simulink model "Full_model_v1"  (R2023b)
settings: Solver=VariableStepAuto  StartTime=0.0  StopTime=simu.duration  FixedStep=simu.timestep  MaxStep=0.1  MinStep=1e-16  RelTol=1e-3
undefined symbols (not defined in the file or in its folder): ptosim, Z_OPT_fixed
libraries: fl_lib x47, nesl_utility x42, ee_lib x11, simulink x1
settings Model: Creator=tedbrekken  LastModifiedBy=inyongkim
settings DebuggingCC: UnconnectedInputMsg=warning  UnconnectedOutputMsg=warning  UnconnectedLineMsg=warning
settings ModelReferenceCC: EnableRefExpFcnMdlSchedulingChecks=on
settings RTWCC: DLArmComputeVersion=19.05

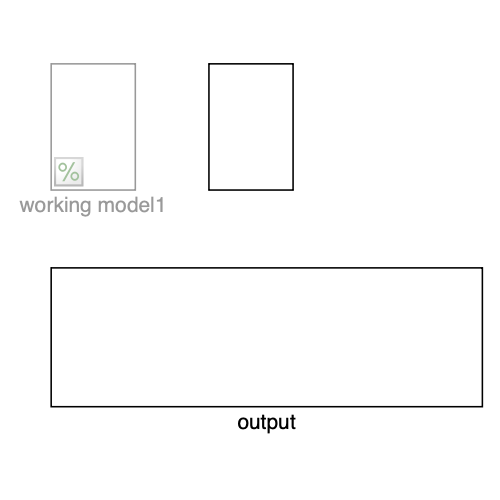
[thumbnail: Simulink's stored preview of the top-level diagram]
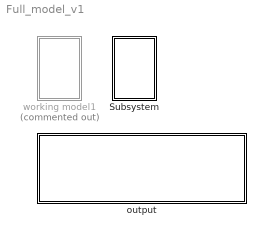
== system Full_model_v1 ==
  Subsystem : Subsystem
  output : Subsystem
  working model1 : Subsystem  Commented=on

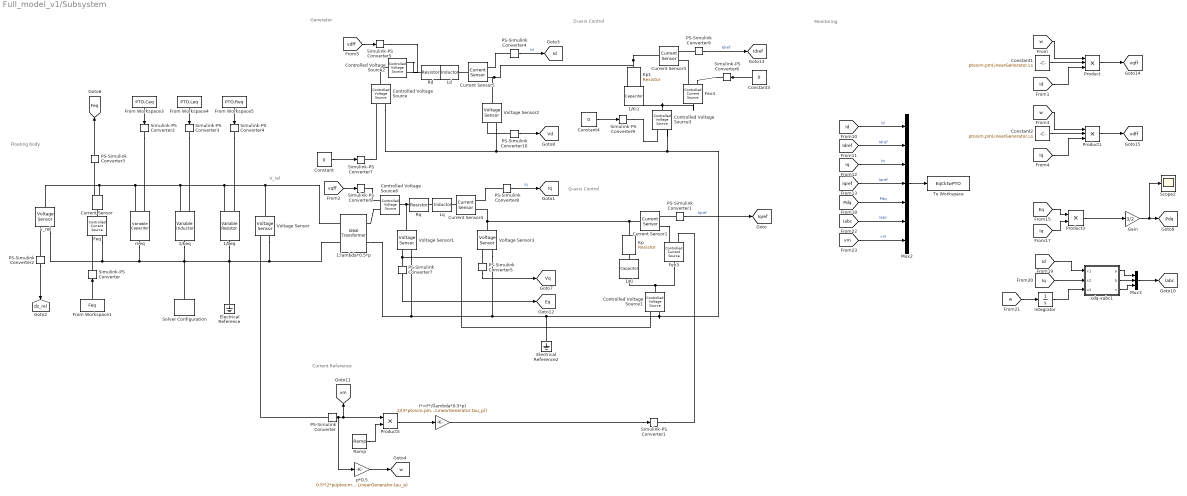
== system Full_model_v1/Subsystem ==
  note: Q-axis Control
  note: Current Reference
  note: Monitoring
  note: Generator
  note: V_rel
  note: D-axis Control
  note: Floating body
  1/Ki : fl_lib/Electrical/Electrical Elements/Capacitor  c=1/(ptosim.pmLinearGenerator.Rs*ptosim.pmLinearGenerator.BWi) F  r=1e-6 Ohm  g=0 1/Ohm  i_specify=off  i_priority=None  i=0 A  i_nominal_specify=off  i_nominal_unit=A  i_nominal_value=1  v_specify=off  v_priority=None  v=0 V  v_nominal_specify=off  v_nominal_unit=V  v_nominal_value=1  vc_specify=off  vc_priority=High  vc=0 V  vc_nominal_specify=off  vc_nominal_unit=V  vc_nominal_value=1
  1/Ki1 : fl_lib/Electrical/Electrical Elements/Capacitor  c=1/(ptosim.pmLinearGenerator.Rs*ptosim.pmLinearGenerator.BWi) F  r=1e-6 Ohm  g=0 1/Ohm  i_specify=off  i_priority=None  i=0 A  i_nominal_specify=off  i_nominal_unit=A  i_nominal_value=1  v_specify=off  v_priority=None  v=0 V  v_nominal_specify=off  v_nominal_unit=V  v_nominal_value=1  vc_specify=off  vc_priority=High  vc=0 V  vc_nominal_specify=off  vc_nominal_unit=V  vc_nominal_value=1
  1/beq : fl_lib/Electrical/Electrical Elements/Variable Resistor  Rmin=0 Ohm  thermalEnable=false  thermal_mass=1 J/K  i_specify=off  i_priority=None  i=0 A  i_nominal_specify=off  i_nominal_unit=A  i_nominal_value=1  v_specify=off  v_priority=None  v=0 V  v_nominal_specify=off  v_nominal_unit=V  v_nominal_value=1  T_specify=off  T_priority=None  T=300 K  T_nominal_specify=off  T_nominal_unit=K  T_nominal_value=1
  1/keq : ee_lib/Passive/Variable Inductor  prm=2  Lmin=1e-8 H  g=0 1/Ohm  i0=0 A  phi0=0 Wb
      settings: InternalSimscapePortConfiguration="{\"Bottom\":[],\"Left\":[{\"id\":\"L\",\"label\":\"L\",\"type\":\"input\"},{\"id\":\"p\",\"label\":\"+\",\"type\":\"foundation.electrical.electrical\"}],\"Right\":[{\"id\":\"n\",\"label\":\"-\",\"type\":\"foundation.electrical.electrical\"}],\"Top\":[]}"
  1:lambda*0.5*p : fl_lib/Electrical/Electrical Elements/Ideal Transformer  n=1/(ptosim.pmLinearGenerator.lambda_fd*0.5*(2*pi/ptosim.pmLinearGenerator.tau_p))  i1_specify=off  i1_priority=None  i1=0 A  i1_nominal_specify=off  i1_nominal_unit=A  i1_nominal_value=1  v1_specify=off  v1_priority=None  v1=0 V  v1_nominal_specify=off  v1_nominal_unit=V  v1_nominal_value=1  i2_specify=off  i2_priority=None  i2=0 A  i2_nominal_specify=off  i2_nominal_unit=A  i2_nominal_value=1  v2_specify=off  v2_priority=None  v2=0 V  v2_nominal_specify=off  v2_nominal_unit=V  v2_nominal_value=1
  Constant : Constant  Value=0
  Constant1 : Constant  Value=ptosim.pmLinearGenerator.Ls
  Constant2 : Constant  Value=ptosim.pmLinearGenerator.Ls
  Constant3 : Constant  Value=0
  Constant4 : Constant  Value=0
  Controlled Voltage Source{,1..3,6} (5 alike) : fl_lib/Electrical/Electrical Sources/Controlled Voltage Source
  Current Sensor{,1,3..5} (5 alike) : fl_lib/Electrical/Electrical Sensors/Current Sensor
  Electrical Reference : fl_lib/Electrical/Electrical Elements/Electrical Reference
  Electrical Reference2 : fl_lib/Electrical/Electrical Elements/Electrical Reference
  Feq : fl_lib/Electrical/Electrical Sources/Controlled Current Source
  Fex3 : fl_lib/Electrical/Electrical Sources/Controlled Current Source
  Fex4 : fl_lib/Electrical/Electrical Sources/Controlled Current Source
  From Workspace1 : FromWorkspace  VariableName=Feq
  From Workspace3 : FromWorkspace  VariableName=PTO.Ceq
  From Workspace4 : FromWorkspace  VariableName=PTO.Leq
  From Workspace5 : FromWorkspace  VariableName=PTO.Req
  Gain : Gain  Gain=3/2
  I*=F*/(lambda*0.5*p) : Gain  Gain=2/(3*ptosim.pmLinearGenerator.lambda_fd*0.5*(2*pi/ptosim.pmLinearGenerator.tau_p))
  Integrator : Integrator
  Kp : fl_lib/Electrical/Electrical Elements/Resistor  R=ptosim.pmLinearGenerator.Ls*ptosim.pmLinearGenerator.BWi Ohm  i_specify=off  i_priority=None  i=0 A  i_nominal_specify=off  i_nominal_unit=A  i_nominal_value=1  v_specify=off  v_priority=None  v=0 V  v_nominal_specify=off  v_nominal_unit=V  v_nominal_value=1
  Kp1 : fl_lib/Electrical/Electrical Elements/Resistor  R=ptosim.pmLinearGenerator.Ls*ptosim.pmLinearGenerator.BWi Ohm  i_specify=off  i_priority=None  i=0 A  i_nominal_specify=off  i_nominal_unit=A  i_nominal_value=1  v_specify=off  v_priority=None  v=0 V  v_nominal_specify=off  v_nominal_unit=V  v_nominal_value=1
  Ld : ee_lib/Passive/Inductor  l=ptosim.pmLinearGenerator.Ls H  enable_L_tol=ee.enum.toleranceApplication.none  L_tol=20  tol_distribution=ee.enum.toleranceDistribution.uniform  nSigma=4  r=0 Ohm  g=1e-9 1/Ohm  enable_operating_limits=ee.enum.enable.no  operating_limit_action=ee.enum.passive.reportOpLim.warn  max_working_current=1 A  power_rating=1 W  enable_faults=ee.enum.enable.no  fault_action=simscape.enum.assert.action.none  lambdaPercent=50  k_faulted=0.9999  turnsShort=ee.enum.passive.inductor.turnsShortOption.no  openCct=ee.enum.enable.no  groundShort=ee.enum.passive.inductor.groundShortOption.no  groundShortG=0 1/Ohm  tau_fault=1e-3 s  fault_trigger=ee.enum.faults.faultTrigger.temporal  t_fault=1 s  max_permissible_voltage=100 V  n_fail_on_voltage=1  max_permissible_current=1 A  t_fail_on_current=1 s  i_L_specify=off  i_L_priority=High  i_L=0 A  i_L_nominal_specify=off  i_L_nominal_unit=A  i_L_nominal_value=1
  Lq : ee_lib/Passive/Inductor  l=ptosim.pmLinearGenerator.Ls H  enable_L_tol=ee.enum.toleranceApplication.none  L_tol=20  tol_distribution=ee.enum.toleranceDistribution.uniform  nSigma=4  r=0 Ohm  g=1e-9 1/Ohm  enable_operating_limits=ee.enum.enable.no  operating_limit_action=ee.enum.passive.reportOpLim.warn  max_working_current=1 A  power_rating=1 W  enable_faults=ee.enum.enable.no  fault_action=simscape.enum.assert.action.none  lambdaPercent=50  k_faulted=0.9999  turnsShort=ee.enum.passive.inductor.turnsShortOption.no  openCct=ee.enum.enable.no  groundShort=ee.enum.passive.inductor.groundShortOption.no  groundShortG=0 1/Ohm  tau_fault=1e-3 s  fault_trigger=ee.enum.faults.faultTrigger.temporal  t_fault=1 s  max_permissible_voltage=100 V  n_fail_on_voltage=1  max_permissible_current=1 A  t_fail_on_current=1 s  i_L_specify=off  i_L_priority=High  i_L=0 A  i_L_nominal_specify=off  i_L_nominal_unit=A  i_L_nominal_value=1
  Mux2 : Mux  Inputs=7
  Mux3 : Mux  Inputs=3
  PS-Simulink Converter{,1,4..5,7..10} (8 alike) : nesl_utility/PS-Simulink Converter  PhysicalDomain=network_engine_domain  SubClassName=ps_output  LeftPortType=input  RightPortType=output  PseudoPeriodic=off  Frequencies=[]  VectorFormat=inherit  Unit=inherit  AffineConversion=off
  PS-Simulink Converter2 : nesl_utility/PS-Simulink Converter  PhysicalDomain=network_engine_domain  SubClassName=ps_output  LeftPortType=input  RightPortType=output  PseudoPeriodic=off  Frequencies=[]  VectorFormat=1-D array  Unit=inherit  AffineConversion=off
  PS-Simulink Converter3 : nesl_utility/PS-Simulink Converter  PhysicalDomain=network_engine_domain  SubClassName=ps_output  LeftPortType=input  RightPortType=output  PseudoPeriodic=off  Frequencies=[]  VectorFormat=1-D array  Unit=inherit  AffineConversion=off
  Product : Product  Inputs=3
  Product1 : Product  Inputs=3
  Product3 : Product
  Product5 : Product
  Ramp : simulink/Sources/Ramp  slope=0.1/(ptosim.pmLinearGenerator.R1+ptosim.pmLinearGenerator.R2)  start=35  InitialOutput=0.1/(ptosim.pmLinearGenerator.R1+ptosim.pmLinearGenerator.R2)
  Rd : fl_lib/Electrical/Electrical Elements/Resistor  R=ptosim.pmLinearGenerator.Rs Ohm  i_specify=off  i_priority=None  i=0 A  i_nominal_specify=off  i_nominal_unit=A  i_nominal_value=1  v_specify=off  v_priority=None  v=0 V  v_nominal_specify=off  v_nominal_unit=V  v_nominal_value=1
  Rq : fl_lib/Electrical/Electrical Elements/Resistor  R=ptosim.pmLinearGenerator.Rs Ohm  i_specify=off  i_priority=None  i=0 A  i_nominal_specify=off  i_nominal_unit=A  i_nominal_value=1  v_specify=off  v_priority=None  v=0 V  v_nominal_specify=off  v_nominal_unit=V  v_nominal_value=1
  Scope2 : Scope
  Simulink-PS Converter{,1..9} (10 alike) : nesl_utility/Simulink-PS Converter  PhysicalDomain=network_engine_domain  SubClassName=ps_input  LeftPortType=input  RightPortType=output  PseudoPeriodic=off  Frequencies=[]  NoiseDistribution=none  NoiseParameters=[]  Unit=1  AffineConversion=off  FilteringAndDerivatives=provide  SimscapeFilterOrder=1  InputFilterTimeConstant=0.001  UdotUserProvided=0
  Solver Configuration : nesl_utility/Solver Configuration  PhysicalDomain=network_engine_domain  SubClassName=solver  LeftPortType=input  RightPortType=generic  Tones=[]  Harmonics=[]  SimulateNoise=off  Profile=off  UseLocalSampling=off  EnableSwitchedLinearOptims=on  FrequencyDomain=off  UseCCode=off  RelTol=0.001  AbsTol=1e-06  MinStep=1e-09  ToWorkspace=off  RevertToSquareIcSolve=off  NumHomotopyIterations=100  PhasorMode=off  PhasorModeNumHarmonics=1  ConsistencySolver=NEWTON_FTOL  IndexReductionMethod=DerivativeReplacement  DoDC=off  ResidualTolerance=1e-09  ConsistencyTolSource=GLOBAL  ConsistencyAbsTol=0.001  ConsistencyRelTol=0.001  ConsistencyTolFactor=0.001  UseLocalSolver=off  LocalSolverChoice=NE_TRAPEZOIDAL_ADVANCER  ResolveIndetEquations=on  FunctionEvalNumThread=1  LocalSolverSampleTime=0.1  DoFixedCost=off  MaxNonlinIter=3  MaxModeIter=2  ComputeImpulses=off  ImpulseIterations=2  LinearAlgebra=auto  LinearAlgebraNumThread=0  EquationFormulation=NE_TIME_EF  DelaysMemoryBudget=1024  AutomaticFiltering=off  FilteringTimeConstant=0.001  PartitionStorageMethod=AS_NEEDED  PartitionMemoryBudget=1024  PartitionMethod=ROBUST  MultibodyUseLocalSolver=off  MultibodyLocalSolverChoice=ODE1  MultibodyLocalSolverSampleTime=0.001
  To Workspace : ToWorkspace  VariableName=EqCktwPTO  SaveFormat=Timeseries  SampleTime=-1
  Voltage Sensor{,1..3} (4 alike) : fl_lib/Electrical/Electrical Sensors/Voltage Sensor
  meq : ee_lib/Passive/Variable Capacitor  prm=2  Cmin=1e-9 F  r=0 Ohm  v0=0 V  q0=0 C
      settings: InternalSimscapePortConfiguration="{\"Bottom\":[],\"Left\":[{\"id\":\"C\",\"label\":\"C\",\"type\":\"input\"},{\"id\":\"p\",\"label\":\"+\",\"type\":\"foundation.electrical.electrical\"}],\"Right\":[{\"id\":\"n\",\"label\":\"-\",\"type\":\"foundation.electrical.electrical\"}],\"Top\":[]}"
  p*0.5 : Gain  Gain=0.5*(2*pi/ptosim.pmLinearGenerator.tau_p)
  v_rel : fl_lib/Electrical/Electrical Sensors/Voltage Sensor
  xdq-xabc1 : MATLAB Function  TreatAsAtomicUnit=on
  tag scope: Eq=global, Feq=global, Iabc=global, Id=global, Idref=global, Iq=global, Iqref=global, Pdq=global, Vd=global, Vq=global, dz_rel=global, vdff=global, vm=global, vqff=global, w=global
  wires:
  From Workspace3/1 -> Simulink-PS Converter2/1
  From Workspace1/1 -> Simulink-PS Converter/1
  PS-Simulink Converter2/1 -> [dz_rel]
  PS-Simulink Converter3/1 -> [Feq]
  From Workspace4/1 -> Simulink-PS Converter3/1
  From Workspace5/1 -> Simulink-PS Converter4/1
  PS-Simulink Converter/1 -> [vm], Product5/1, p*0.5/1
  [vqff] -> Simulink-PS Converter8/1
  [vdff] -> Simulink-PS Converter5/1
  PS-Simulink Converter7/1 -> [Eq]
  Ramp/1 -> Product5/2
  PS-Simulink Converter9/1 -> [Idref]  "Idref"
  Constant3/1 -> Simulink-PS Converter6/1
  PS-Simulink Converter1/1 -> [Iqref]  "Iqref"
  PS-Simulink Converter4/1 -> [Id]  "Id"
  Product5/1 -> I*=F*/(lambda*0.5*p)/1
  Constant/1 -> Simulink-PS Converter7/1
  PS-Simulink Converter10/1 -> [Vd]
  PS-Simulink Converter8/1 -> [Iq]  "Iq"
  I*=F*/(lambda*0.5*p)/1 -> Simulink-PS Converter1/1
  p*0.5/1 -> [w]
  PS-Simulink Converter5/1 -> [Vq]
  [Idref] -> Mux2/2  "Idref"
  [Iabc] -> Mux2/6  "Iabc"
  [Eq] -> Product3/1
  xdq-xabc1/3(c) -> Mux3/3
  Gain/1 -> Scope2/1, [Pdq]
  [Iqref] -> Mux2/4  "Iqref"
  Product3/1 -> Gain/1
  [w] -> Product1/1
  [Iq] -> Mux2/3  "Iq"
  [Iq] -> Product1/3
  Product/1 -> [vqff]
  xdq-xabc1/1(a) -> Mux3/1
  [Id] -> Product/3
  [Pdq] -> Mux2/5  "Pdq"
  xdq-xabc1/2(b) -> Mux3/2
  Mux3/1 -> [Iabc]
  [Id] -> xdq-xabc1/1(x1)
  [w] -> Product/1
  [Id] -> Mux2/1  "Id"
  Mux2/1 -> To Workspace/1
  Product1/1 -> [vdff]
  [Iq] -> Product3/2
  Integrator/1 -> xdq-xabc1/3(u1)
  [vm] -> Mux2/7  "vm"
  [Iq] -> xdq-xabc1/2(x2)
  Constant1/1 -> Product/2
  Constant2/1 -> Product1/2
  [w] -> Integrator/1
  Constant4/1 -> Simulink-PS Converter9/1
  connections:
  Current Sensor/RConn1 -- PS-Simulink Converter3/LConn1
  PS-Simulink Converter2/LConn1 -- v_rel/RConn1
  Simulink-PS Converter4/RConn1 -- 1/beq/LConn1
  Simulink-PS Converter/RConn1 -- Feq/RConn1
  Simulink-PS Converter3/RConn1 -- 1/keq/LConn1
  Voltage Sensor/LConn1 -- 1:lambda*0.5*p/LConn1 -- 1/beq/LConn2 -- Current Sensor/RConn2 -- v_rel/LConn1 -- meq/LConn2 -- 1/keq/LConn2
  Simulink-PS Converter2/RConn1 -- meq/LConn1
  Electrical Reference/LConn1 -- Solver Configuration/RConn1 -- v_rel/RConn2 -- Feq/RConn2 -- meq/RConn1 -- 1/keq/RConn1 -- 1:lambda*0.5*p/LConn2 -- Voltage Sensor/RConn2 -- 1/beq/RConn1
  Feq/LConn1 -- Current Sensor/LConn1
  PS-Simulink Converter7/LConn1 -- Controlled Voltage Source1/RConn1 -- Voltage Sensor1/RConn1
  PS-Simulink Converter9/LConn1 -- Current Sensor3/RConn1
  Voltage Sensor2/RConn2 -- Electrical Reference2/LConn1 -- Voltage Sensor3/RConn2 -- Voltage Sensor1/RConn2 -- 1:lambda*0.5*p/RConn2 -- Controlled Voltage Source1/RConn2 -- Controlled Voltage Source3/RConn2 -- Controlled Voltage Source/RConn2
  PS-Simulink Converter/LConn1 -- Voltage Sensor/RConn1
  Controlled Voltage Source6/LConn1 -- Voltage Sensor1/LConn1 -- Rq/LConn1
  Controlled Voltage Source2/LConn1 -- Controlled Voltage Source/LConn1
  Kp/LConn1 -- Current Sensor4/RConn2 -- Voltage Sensor3/LConn1 -- Current Sensor1/LConn1
  Kp1/LConn1 -- Voltage Sensor2/LConn1 -- Current Sensor5/RConn2 -- Current Sensor3/LConn1
  Rq/RConn1 -- Lq/LConn1
  Controlled Voltage Source3/LConn1 -- 1/Ki1/RConn1 -- Fex4/LConn1
  PS-Simulink Converter4/LConn1 -- Current Sensor5/RConn1
  PS-Simulink Converter1/LConn1 -- Current Sensor1/RConn1
  Simulink-PS Converter1/RConn1 -- Fex3/RConn1
  Simulink-PS Converter7/RConn1 -- Controlled Voltage Source/RConn1
  Simulink-PS Converter8/RConn1 -- Controlled Voltage Source6/RConn1
  Rd/RConn1 -- Ld/LConn1
  1/Ki/LConn1 -- Kp/RConn1
  PS-Simulink Converter8/LConn1 -- Current Sensor4/RConn1
  Current Sensor1/RConn2 -- Fex3/RConn2
  Controlled Voltage Source1/LConn1 -- 1/Ki/RConn1 -- Fex3/LConn1
  Current Sensor5/LConn1 -- Ld/RConn1
  PS-Simulink Converter5/LConn1 -- Voltage Sensor3/RConn1
  Current Sensor4/LConn1 -- Lq/RConn1
  Fex4/RConn2 -- Current Sensor3/RConn2
  1/Ki1/LConn1 -- Kp1/RConn1
  Simulink-PS Converter5/RConn1 -- Controlled Voltage Source2/RConn1
  Controlled Voltage Source2/RConn2 -- Rd/LConn1
  Simulink-PS Converter6/RConn1 -- Fex4/RConn1
  Controlled Voltage Source6/RConn2 -- 1:lambda*0.5*p/RConn1
  PS-Simulink Converter10/LConn1 -- Voltage Sensor2/RConn1
  Simulink-PS Converter9/RConn1 -- Controlled Voltage Source3/RConn1

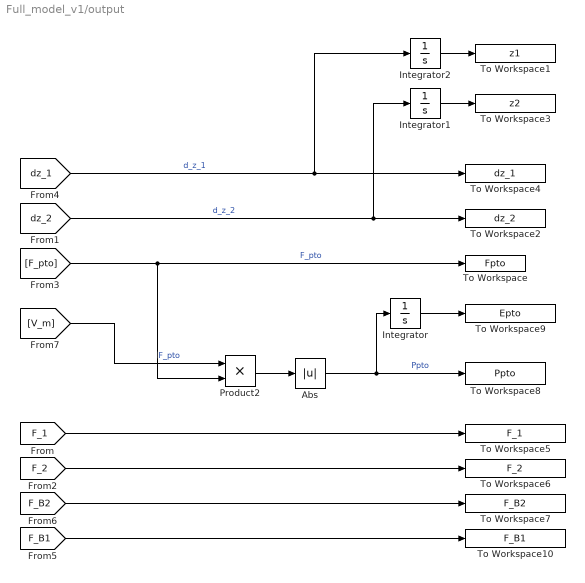
== system Full_model_v1/output ==
  Abs : Abs  SaturateOnIntegerOverflow=off
  Integrator : Integrator
  Integrator1 : Integrator
  Integrator2 : Integrator
  Product2 : Product
  To Workspace : ToWorkspace  VariableName=Fpto  SaveFormat=Timeseries  SampleTime=-1
  To Workspace1 : ToWorkspace  VariableName=z1  SaveFormat=Timeseries  SampleTime=-1
  To Workspace10 : ToWorkspace  VariableName=F_B1  SaveFormat=Timeseries  SampleTime=-1
  To Workspace2 : ToWorkspace  VariableName=dz_2  SaveFormat=Timeseries  SampleTime=-1
  To Workspace3 : ToWorkspace  VariableName=z2  SaveFormat=Timeseries  SampleTime=-1
  To Workspace4 : ToWorkspace  VariableName=dz_1  SaveFormat=Timeseries  SampleTime=-1
  To Workspace5 : ToWorkspace  VariableName=F_1  SaveFormat=Timeseries  SampleTime=-1
  To Workspace6 : ToWorkspace  VariableName=F_2  SaveFormat=Timeseries  SampleTime=-1
  To Workspace7 : ToWorkspace  VariableName=F_B2  SaveFormat=Timeseries  SampleTime=-1
  To Workspace8 : ToWorkspace  VariableName=Ppto  SaveFormat=Timeseries  SampleTime=-1
  To Workspace9 : ToWorkspace  VariableName=Epto  SaveFormat=Timeseries  SampleTime=-1
  wires:
  Integrator/1 -> To Workspace9/1
  [dz_1] -> Integrator2/1, To Workspace4/1  "d_z_1"
  [F_pto] -> To Workspace/1, Product2/2  "F_pto"
  Abs/1 -> To Workspace8/1, Integrator/1  "Ppto"
  Product2/1 -> Abs/1
  [dz_2] -> Integrator1/1, To Workspace2/1  "d_z_2"
  [F_1] -> To Workspace5/1
  [F_2] -> To Workspace6/1
  [F_B2] -> To Workspace7/1
  [F_B1] -> To Workspace10/1
  [V_m] -> Product2/1  "F_pto"
  Integrator2/1 -> To Workspace1/1
  Integrator1/1 -> To Workspace3/1

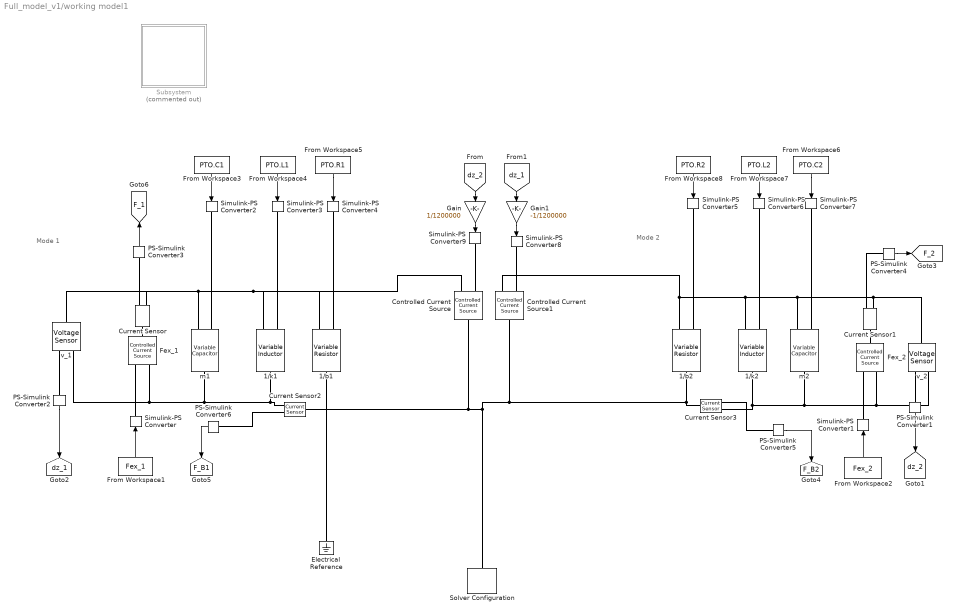
== system Full_model_v1/working model1 ==
  note: Mode 1
  note: Mode 2
  1/b1 : fl_lib/Electrical/Electrical Elements/Variable Resistor  Rmin=0 Ohm  thermalEnable=false  thermal_mass=1 J/K  i_specify=off  i_priority=None  i=0 A  i_nominal_specify=off  i_nominal_unit=A  i_nominal_value=1  v_specify=off  v_priority=None  v=0 V  v_nominal_specify=off  v_nominal_unit=V  v_nominal_value=1  T_specify=off  T_priority=None  T=300 K  T_nominal_specify=off  T_nominal_unit=K  T_nominal_value=1
  1/b2 : fl_lib/Electrical/Electrical Elements/Variable Resistor  Rmin=0 Ohm  thermalEnable=false  thermal_mass=1 J/K  i_specify=off  i_priority=None  i=0 A  i_nominal_specify=off  i_nominal_unit=A  i_nominal_value=1  v_specify=off  v_priority=None  v=0 V  v_nominal_specify=off  v_nominal_unit=V  v_nominal_value=1  T_specify=off  T_priority=None  T=300 K  T_nominal_specify=off  T_nominal_unit=K  T_nominal_value=1
  1/k1 : ee_lib/Passive/Variable Inductor  prm=2  Lmin=1e-8 H  g=0 1/Ohm  i0=0 A  phi0=0 Wb
      settings: InternalSimscapePortConfiguration="{\"Bottom\":[],\"Left\":[{\"id\":\"L\",\"label\":\"L\",\"type\":\"input\"},{\"id\":\"p\",\"label\":\"+\",\"type\":\"foundation.electrical.electrical\"}],\"Right\":[{\"id\":\"n\",\"label\":\"-\",\"type\":\"foundation.electrical.electrical\"}],\"Top\":[]}"
  1/k2 : ee_lib/Passive/Variable Inductor  prm=2  Lmin=1e-8 H  g=0 1/Ohm  i0=0 A  phi0=0 Wb
      settings: InternalSimscapePortConfiguration="{\"Bottom\":[],\"Left\":[{\"id\":\"L\",\"label\":\"L\",\"type\":\"input\"},{\"id\":\"p\",\"label\":\"+\",\"type\":\"foundation.electrical.electrical\"}],\"Right\":[{\"id\":\"n\",\"label\":\"-\",\"type\":\"foundation.electrical.electrical\"}],\"Top\":[]}"
  Controlled Current Source : fl_lib/Electrical/Electrical Sources/Controlled Current Source
  Controlled Current Source1 : fl_lib/Electrical/Electrical Sources/Controlled Current Source
  Current Sensor{,1..3} (4 alike) : fl_lib/Electrical/Electrical Sensors/Current Sensor
  Electrical Reference : fl_lib/Electrical/Electrical Elements/Electrical Reference
  Fex_1 : fl_lib/Electrical/Electrical Sources/Controlled Current Source
  Fex_2 : fl_lib/Electrical/Electrical Sources/Controlled Current Source
  From Workspace1 : FromWorkspace  VariableName=Fex_1
  From Workspace2 : FromWorkspace  VariableName=Fex_2
  From Workspace3 : FromWorkspace  VariableName=PTO.C1
  From Workspace4 : FromWorkspace  VariableName=PTO.L1
  From Workspace5 : FromWorkspace  VariableName=PTO.R1
  From Workspace6 : FromWorkspace  VariableName=PTO.C2
  From Workspace7 : FromWorkspace  VariableName=PTO.L2
  From Workspace8 : FromWorkspace  VariableName=PTO.R2
  Gain : Gain  Gain=1/1200000
  Gain1 : Gain  Gain=-1/1200000
  PS-Simulink Converter{1..6} (6 alike) : nesl_utility/PS-Simulink Converter  PhysicalDomain=network_engine_domain  SubClassName=ps_output  LeftPortType=input  RightPortType=output  PseudoPeriodic=off  Frequencies=[]  VectorFormat=1-D array  Unit=inherit  AffineConversion=off
  Simulink-PS Converter{,1..9} (10 alike) : nesl_utility/Simulink-PS Converter  PhysicalDomain=network_engine_domain  SubClassName=ps_input  LeftPortType=input  RightPortType=output  PseudoPeriodic=off  Frequencies=[]  NoiseDistribution=none  NoiseParameters=[]  Unit=1  AffineConversion=off  FilteringAndDerivatives=provide  SimscapeFilterOrder=1  InputFilterTimeConstant=0.001  UdotUserProvided=0
  Solver Configuration : nesl_utility/Solver Configuration  PhysicalDomain=network_engine_domain  SubClassName=solver  LeftPortType=input  RightPortType=generic  Tones=[]  Harmonics=[]  SimulateNoise=off  Profile=off  UseLocalSampling=off  EnableSwitchedLinearOptims=on  FrequencyDomain=off  UseCCode=off  RelTol=0.001  AbsTol=1e-06  MinStep=1e-09  ToWorkspace=off  RevertToSquareIcSolve=off  NumHomotopyIterations=100  PhasorMode=off  PhasorModeNumHarmonics=1  ConsistencySolver=NEWTON_FTOL  IndexReductionMethod=DerivativeReplacement  DoDC=off  ResidualTolerance=1e-09  ConsistencyTolSource=GLOBAL  ConsistencyAbsTol=0.001  ConsistencyRelTol=0.001  ConsistencyTolFactor=0.001  UseLocalSolver=off  LocalSolverChoice=NE_TRAPEZOIDAL_ADVANCER  ResolveIndetEquations=on  FunctionEvalNumThread=1  LocalSolverSampleTime=0.1  DoFixedCost=off  MaxNonlinIter=3  MaxModeIter=2  ComputeImpulses=off  ImpulseIterations=2  LinearAlgebra=auto  LinearAlgebraNumThread=0  EquationFormulation=NE_TIME_EF  DelaysMemoryBudget=1024  AutomaticFiltering=off  FilteringTimeConstant=0.001  PartitionStorageMethod=AS_NEEDED  PartitionMemoryBudget=1024  PartitionMethod=ROBUST  MultibodyUseLocalSolver=off  MultibodyLocalSolverChoice=ODE1  MultibodyLocalSolverSampleTime=0.001
  Subsystem : Subsystem  Commented=on
  m1 : ee_lib/Passive/Variable Capacitor  prm=2  Cmin=1e-9 F  r=0 Ohm  v0=0 V  q0=0 C
      settings: InternalSimscapePortConfiguration="{\"Bottom\":[],\"Left\":[{\"id\":\"C\",\"label\":\"C\",\"type\":\"input\"},{\"id\":\"p\",\"label\":\"+\",\"type\":\"foundation.electrical.electrical\"}],\"Right\":[{\"id\":\"n\",\"label\":\"-\",\"type\":\"foundation.electrical.electrical\"}],\"Top\":[]}"
  m2 : ee_lib/Passive/Variable Capacitor  prm=2  Cmin=1e-9 F  r=0 Ohm  v0=0 V  q0=0 C
      settings: InternalSimscapePortConfiguration="{\"Bottom\":[],\"Left\":[{\"id\":\"C\",\"label\":\"C\",\"type\":\"input\"},{\"id\":\"p\",\"label\":\"+\",\"type\":\"foundation.electrical.electrical\"}],\"Right\":[{\"id\":\"n\",\"label\":\"-\",\"type\":\"foundation.electrical.electrical\"}],\"Top\":[]}"
  v_1 : fl_lib/Electrical/Electrical Sensors/Voltage Sensor
  v_2 : fl_lib/Electrical/Electrical Sensors/Voltage Sensor
  tag scope: F_1=global, F_2=global, F_B1=global, F_B2=global, dz_1=global, dz_2=global
  wires:
  From Workspace1/1 -> Simulink-PS Converter/1
  PS-Simulink Converter3/1 -> [F_1]
  PS-Simulink Converter2/1 -> [dz_1]
  From Workspace2/1 -> Simulink-PS Converter1/1
  PS-Simulink Converter4/1 -> [F_2]
  PS-Simulink Converter1/1 -> [dz_2]
  PS-Simulink Converter5/1 -> [F_B2]
  PS-Simulink Converter6/1 -> [F_B1]
  From Workspace3/1 -> Simulink-PS Converter2/1
  From Workspace4/1 -> Simulink-PS Converter3/1
  From Workspace5/1 -> Simulink-PS Converter4/1
  From Workspace8/1 -> Simulink-PS Converter5/1
  From Workspace7/1 -> Simulink-PS Converter6/1
  From Workspace6/1 -> Simulink-PS Converter7/1
  Gain1/1 -> Simulink-PS Converter8/1
  [dz_1] -> Gain1/1
  Gain/1 -> Simulink-PS Converter9/1
  [dz_2] -> Gain/1
  connections:
  Fex_2/LConn1 -- Current Sensor1/LConn1
  Current Sensor/LConn1 -- Fex_1/LConn1
  Fex_2/RConn1 -- Simulink-PS Converter1/RConn1
  PS-Simulink Converter1/LConn1 -- v_2/RConn1
  Fex_1/RConn1 -- Simulink-PS Converter/RConn1
  PS-Simulink Converter2/LConn1 -- v_1/RConn1
  Current Sensor1/RConn1 -- PS-Simulink Converter4/LConn1
  Current Sensor/RConn1 -- PS-Simulink Converter3/LConn1
  Fex_1/RConn2 -- m1/RConn1 -- Current Sensor2/RConn2 -- 1/k1/RConn1 -- v_1/RConn2
  Current Sensor2/RConn1 -- PS-Simulink Converter6/LConn1
  Current Sensor3/RConn1 -- PS-Simulink Converter5/LConn1
  Current Sensor3/RConn2 -- 1/k2/RConn1 -- m2/RConn1 -- v_2/RConn2 -- Fex_2/RConn2
  Controlled Current Source/LConn1 -- 1/b1/RConn1 -- Electrical Reference/LConn1 -- Current Sensor2/LConn1 -- Solver Configuration/RConn1 -- Current Sensor3/LConn1 -- 1/b2/RConn1 -- Controlled Current Source1/LConn1
  Simulink-PS Converter2/RConn1 -- m1/LConn1
  Simulink-PS Converter3/RConn1 -- 1/k1/LConn1
  Simulink-PS Converter4/RConn1 -- 1/b1/LConn1
  Simulink-PS Converter5/RConn1 -- 1/b2/LConn1
  Simulink-PS Converter6/RConn1 -- 1/k2/LConn1
  Simulink-PS Converter7/RConn1 -- m2/LConn1
  Controlled Current Source/RConn2 -- 1/b1/LConn2 -- 1/k1/LConn2 -- v_1/LConn1 -- Current Sensor/RConn2 -- m1/LConn2
  v_2/LConn1 -- Controlled Current Source1/RConn2 -- 1/b2/LConn2 -- 1/k2/LConn2 -- m2/LConn2 -- Current Sensor1/RConn2
  Simulink-PS Converter9/RConn1 -- Controlled Current Source/RConn1
  Simulink-PS Converter8/RConn1 -- Controlled Current Source1/RConn1

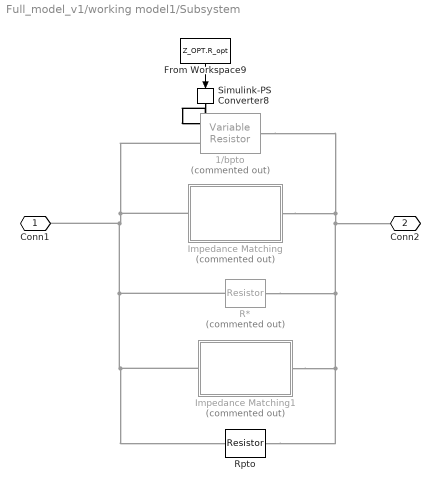
== system Full_model_v1/working model1/Subsystem ==
  1/bpto : fl_lib/Electrical/Electrical Elements/Variable Resistor  Commented=on  Rmin=0 Ohm  thermalEnable=false  thermal_mass=1 J/K  i_specify=off  i_priority=None  i=0 A  i_nominal_specify=off  i_nominal_unit=A  i_nominal_value=1  v_specify=off  v_priority=None  v=0 V  v_nominal_specify=off  v_nominal_unit=V  v_nominal_value=1  T_specify=off  T_priority=None  T=300 K  T_nominal_specify=off  T_nominal_unit=K  T_nominal_value=1
  From Workspace9 : FromWorkspace  VariableName=Z_OPT.R_opt
  Impedance Matching : Subsystem  Commented=on
  Impedance Matching1 : Subsystem  Commented=on
  R* : fl_lib/Electrical/Electrical Elements/Resistor  Commented=on  R=Z_OPT_fixed.R_opt Ohm  i_specify=off  i_priority=None  i=0 A  i_nominal_specify=off  i_nominal_unit=A  i_nominal_value=1  v_specify=off  v_priority=None  v=0 V  v_nominal_specify=off  v_nominal_unit=V  v_nominal_value=1
  Rpto : fl_lib/Electrical/Electrical Elements/Resistor  R=1/1200000 Ohm  i_specify=off  i_priority=None  i=0 A  i_nominal_specify=off  i_nominal_unit=A  i_nominal_value=1  v_specify=off  v_priority=None  v=0 V  v_nominal_specify=off  v_nominal_unit=V  v_nominal_value=1
  Simulink-PS Converter8 : nesl_utility/Simulink-PS Converter  PhysicalDomain=network_engine_domain  SubClassName=ps_input  LeftPortType=input  RightPortType=output  PseudoPeriodic=off  Frequencies=[]  NoiseDistribution=none  NoiseParameters=[]  Unit=1  AffineConversion=off  FilteringAndDerivatives=provide  SimscapeFilterOrder=1  InputFilterTimeConstant=0.001  UdotUserProvided=0
  Conn1 : PMIOPort  Side=Left
  Conn2 : PMIOPort  Port=2  Side=Right
  wires:
  From Workspace9/1 -> Simulink-PS Converter8/1
  connections:
  1/bpto/RConn1 -- Impedance Matching/RConn1 -- Rpto/RConn1 -- Impedance Matching1/RConn1 -- R*/RConn1 -- Conn2/RConn1
  Simulink-PS Converter8/RConn1 -- 1/bpto/LConn1
  1/bpto/LConn2 -- Impedance Matching/LConn1 -- Rpto/LConn1 -- Impedance Matching1/LConn1 -- R*/LConn1 -- Conn1/RConn1

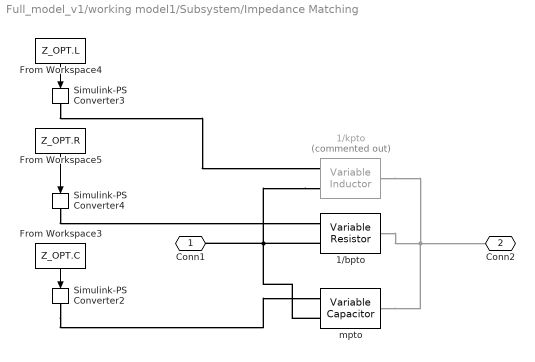
== system Full_model_v1/working model1/Subsystem/Impedance Matching ==
  1/bpto : fl_lib/Electrical/Electrical Elements/Variable Resistor  Rmin=0 Ohm  thermalEnable=false  thermal_mass=1 J/K  i_specify=off  i_priority=None  i=0 A  i_nominal_specify=off  i_nominal_unit=A  i_nominal_value=1  v_specify=off  v_priority=None  v=0 V  v_nominal_specify=off  v_nominal_unit=V  v_nominal_value=1  T_specify=off  T_priority=None  T=300 K  T_nominal_specify=off  T_nominal_unit=K  T_nominal_value=1
  1/kpto : ee_lib/Passive/Variable Inductor  Commented=on  prm=2  Lmin=1e-8 H  g=0 1/Ohm  i0=0 A  phi0=0 Wb
      settings: InternalSimscapePortConfiguration="{\"Bottom\":[],\"Left\":[{\"id\":\"L\",\"label\":\"L\",\"type\":\"input\"},{\"id\":\"p\",\"label\":\"+\",\"type\":\"foundation.electrical.electrical\"}],\"Right\":[{\"id\":\"n\",\"label\":\"-\",\"type\":\"foundation.electrical.electrical\"}],\"Top\":[]}"
  From Workspace3 : FromWorkspace  VariableName=Z_OPT.C
  From Workspace4 : FromWorkspace  VariableName=Z_OPT.L
  From Workspace5 : FromWorkspace  VariableName=Z_OPT.R
  Simulink-PS Converter2 : nesl_utility/Simulink-PS Converter  PhysicalDomain=network_engine_domain  SubClassName=ps_input  LeftPortType=input  RightPortType=output  PseudoPeriodic=off  Frequencies=[]  NoiseDistribution=none  NoiseParameters=[]  Unit=1  AffineConversion=off  FilteringAndDerivatives=provide  SimscapeFilterOrder=1  InputFilterTimeConstant=0.001  UdotUserProvided=0
  Simulink-PS Converter3 : nesl_utility/Simulink-PS Converter  PhysicalDomain=network_engine_domain  SubClassName=ps_input  LeftPortType=input  RightPortType=output  PseudoPeriodic=off  Frequencies=[]  NoiseDistribution=none  NoiseParameters=[]  Unit=1  AffineConversion=off  FilteringAndDerivatives=provide  SimscapeFilterOrder=1  InputFilterTimeConstant=0.001  UdotUserProvided=0
  Simulink-PS Converter4 : nesl_utility/Simulink-PS Converter  PhysicalDomain=network_engine_domain  SubClassName=ps_input  LeftPortType=input  RightPortType=output  PseudoPeriodic=off  Frequencies=[]  NoiseDistribution=none  NoiseParameters=[]  Unit=1  AffineConversion=off  FilteringAndDerivatives=provide  SimscapeFilterOrder=1  InputFilterTimeConstant=0.001  UdotUserProvided=0
  mpto : ee_lib/Passive/Variable Capacitor  prm=2  Cmin=1e-9 F  r=0 Ohm  v0=0 V  q0=0 C
      settings: InternalSimscapePortConfiguration="{\"Bottom\":[],\"Left\":[{\"id\":\"C\",\"label\":\"C\",\"type\":\"input\"},{\"id\":\"p\",\"label\":\"+\",\"type\":\"foundation.electrical.electrical\"}],\"Right\":[{\"id\":\"n\",\"label\":\"-\",\"type\":\"foundation.electrical.electrical\"}],\"Top\":[]}"
  Conn1 : PMIOPort  Side=Left
  Conn2 : PMIOPort  Port=2  Side=Right
  wires:
  From Workspace5/1 -> Simulink-PS Converter4/1
  From Workspace4/1 -> Simulink-PS Converter3/1
  From Workspace3/1 -> Simulink-PS Converter2/1
  connections:
  1/kpto/RConn1 -- 1/bpto/RConn1 -- mpto/RConn1 -- Conn2/RConn1
  Simulink-PS Converter4/RConn1 -- 1/bpto/LConn1
  Simulink-PS Converter3/RConn1 -- 1/kpto/LConn1
  Simulink-PS Converter2/RConn1 -- mpto/LConn1
  1/kpto/LConn2 -- mpto/LConn2 -- Conn1/RConn1 -- 1/bpto/LConn2

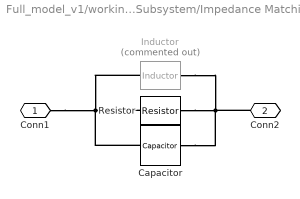
== system Full_model_v1/working model1/Subsystem/Impedance Matching1 ==
  Capacitor : fl_lib/Electrical/Electrical Elements/Capacitor  c=Z_OPT_fixed.C_pto F  r=0 Ohm  g=0 1/Ohm  i_specify=off  i_priority=None  i=0 A  i_nominal_specify=off  i_nominal_unit=A  i_nominal_value=1  v_specify=off  v_priority=None  v=0 V  v_nominal_specify=off  v_nominal_unit=V  v_nominal_value=1  vc_specify=off  vc_priority=High  vc=0 V  vc_nominal_specify=off  vc_nominal_unit=V  vc_nominal_value=1
  Inductor : ee_lib/Passive/Inductor  Commented=on  l=Z_OPT_fixed.L_pto H  enable_L_tol=0  L_tol=20  tol_distribution=1  nSigma=4  r=0 Ohm  g=0 1/Ohm  enable_operating_limits=0  operating_limit_action=2  max_working_current=1 A  power_rating=1 W  enable_faults=ee.enum.enable.no  fault_action=simscape.enum.assert.action.none  lambdaPercent=50  k_faulted=0.9999  turnsShort=0  openCct=0  groundShort=0  groundShortG=0 1/Ohm  tau_fault=1e-3 s  fault_trigger=ee.enum.faults.faultTrigger.temporal  t_fault=1 s  max_permissible_voltage=100 V  n_fail_on_voltage=1  max_permissible_current=1 A  t_fail_on_current=1 s  i_L_specify=off  i_L_priority=High  i_L=0 A  i_L_nominal_specify=off  i_L_nominal_unit=A  i_L_nominal_value=1
  Resistor : fl_lib/Electrical/Electrical Elements/Resistor  R=Z_OPT_fixed.R_pto Ohm  i_specify=off  i_priority=None  i=0 A  i_nominal_specify=off  i_nominal_unit=A  i_nominal_value=1  v_specify=off  v_priority=None  v=0 V  v_nominal_specify=off  v_nominal_unit=V  v_nominal_value=1
  Conn1 : PMIOPort  Side=Left
  Conn2 : PMIOPort  Port=2  Side=Right
  connections:
  Capacitor/LConn1 -- Resistor/LConn1 -- Inductor/LConn1 -- Conn1/RConn1
  Capacitor/RConn1 -- Resistor/RConn1 -- Inductor/RConn1 -- Conn2/RConn1

== matlab function Full_model_v1/Subsystem/xdq-xabc1 ==
  data: x1 input size=1; a output size=1; b output; x2 input; u1 input; c output

function [a,b,c] = fcn(x1,x2,u1)
a = sqrt(2/3)* (sin(u1 + pi/2)*(x1) + cos(u1 + pi/2)*(x2));
b =  sqrt(2/3)*(sin(u1-(2*pi/3)+ pi/2)*(x1) + cos(u1-(2*pi/3)+ pi/2)*(x2));
c =  sqrt(2/3)*(sin(u1+(2*pi/3)+ pi/2)*(x1) + cos(u1+(2*pi/3)+ pi/2)*(x2));
